simulink model "LiniarModel"  (R2023a)
settings: Solver=FixedStepAuto  StartTime=0.0  StopTime=run_time  FixedStep=.001  RelTol=1e-3
values from neighbouring files (symbols this model uses):
  c = 10    [PreLab.m]    (also in PreLab_for_lab.m)
  g = 9.81    [PreLab.m]    (also in PreLab_for_lab.m)
  l = 0.35    [PreLab.m]    (also in PreLab_for_lab.m)
  m = 0.04    [PreLab.m]    (also in PreLab_for_lab.m)
  Myu_d = 1.3*10^(-4)    (= 0.00013)    [PreLab.m]    (also in PreLab_for_lab.m)
  Myu_v = 6.7*10^(-5)    (= 6.7e-05)    [PreLab.m]    (also in PreLab_for_lab.m)
  theta_0 = initial_theta_rad(i)    [PreLab.m]    (also in PreLab_for_lab.m)
  theta_dot_0 = 0    [PreLab.m]    (also in PreLab_for_lab.m)
settings Model: Creator=אלמוג  LastModifiedBy=אלמוג

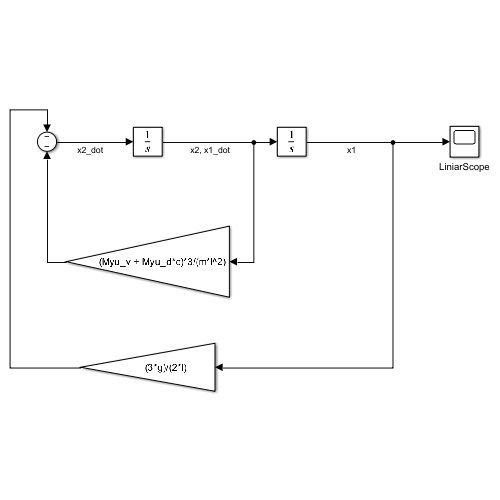
[thumbnail: Simulink's stored preview of the top-level diagram]
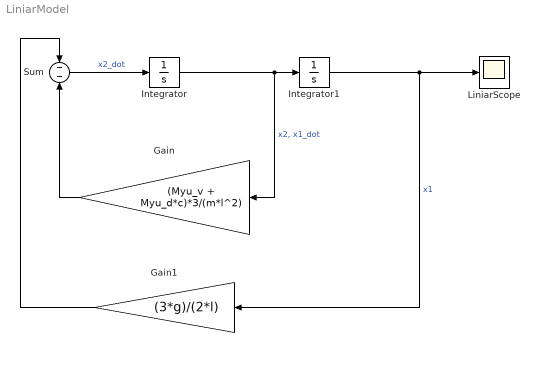
== system LiniarModel ==
  Gain : Gain  Gain=(Myu_v + Myu_d*c)*3/(m*l^2)
  Gain1 : Gain  Gain=(3*g)/(2*l)
  Integrator : Integrator  InitialCondition=theta_dot_0
  Integrator1 : Integrator  InitialCondition=theta_0
  LiniarScope : Scope
  Sum : Sum  Inputs=--
  wires:
  Integrator1/1 -> Gain1/1, LiniarScope/1  "x1"
  Gain1/1 -> Sum/1
  Sum/1 -> Integrator/1  "x2_dot"
  Integrator/1 -> Gain/1, Integrator1/1  "x2, x1_dot"
  Gain/1 -> Sum/2
